simulink model "Simul_ContPID"  (R2024b)
settings: Solver=VariableStepAuto  StartTime=0.0  StopTime=6  RelTol=1e-3
undefined symbols (not defined in the file): Kp, Kpe, T, Te, Ti
settings Model: Creator=Celso  LastModifiedBy=syaba

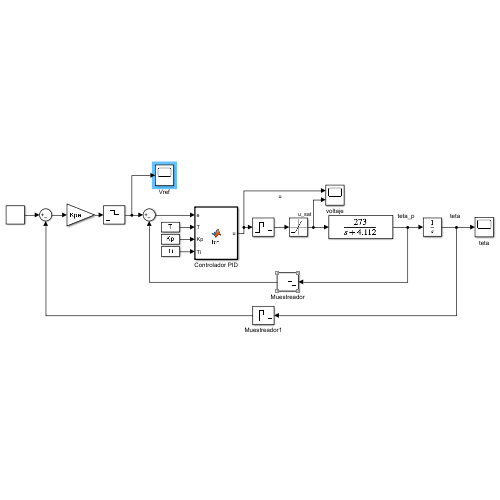
[thumbnail: Simulink's stored preview of the top-level diagram]
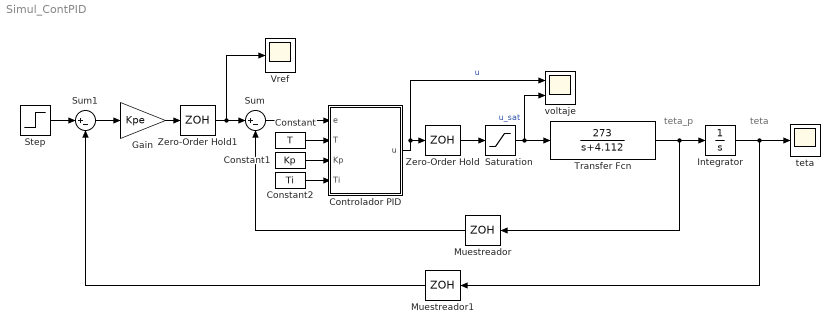
== system Simul_ContPID ==
  note: teta
  note: teta_p
  Constant : Constant  Value=T
  Constant1 : Constant  Value=Kp
  Constant2 : Constant  Value=Ti
  Controlador PID : MATLAB Function  TreatAsAtomicUnit=on  SystemSampleTime=T
  Gain : Gain  Gain=Kpe
  Integrator : Integrator
  Muestreador : ZeroOrderHold  SampleTime=T
  Muestreador1 : ZeroOrderHold  SampleTime=Te
  Saturation : Saturate  UpperLimit=3  LowerLimit=-3
  Step : Step  Time=0  After=100  SampleTime=0
  Sum : Sum  Inputs=|+-
  Sum1 : Sum  Inputs=|+-
  Transfer Fcn : TransferFcn  Numerator=[273]  Denominator=[1 4.112]
  Vref : Scope
  Zero-Order Hold : ZeroOrderHold  SampleTime=T
  Zero-Order Hold1 : ZeroOrderHold  SampleTime=Te
  teta : Scope
  voltaje : Scope  NumInputPorts=2
  wires:
  Constant/1 -> Controlador PID/2(T)
  Sum/1 -> Controlador PID/1(e)
  Controlador PID/1(u) -> voltaje/1, Zero-Order Hold/1  "u"
  Transfer Fcn/1 -> Integrator/1, Muestreador/1
  Muestreador/1 -> Sum/2
  Zero-Order Hold/1 -> Saturation/1
  Saturation/1 -> voltaje/2, Transfer Fcn/1  "u_sat"
  Constant1/1 -> Controlador PID/3(Kp)
  Constant2/1 -> Controlador PID/4(Ti)
  Gain/1 -> Zero-Order Hold1/1
  Zero-Order Hold1/1 -> Vref/1, Sum/1
  Integrator/1 -> teta/1, Muestreador1/1
  Muestreador1/1 -> Sum1/2
  Sum1/1 -> Gain/1
  Step/1 -> Sum1/1

== matlab function Simul_ContPID/Controlador PID ==
  data: e input; u output; T input; Kp input; Ti input
function u = fcn(e,T, Kp, Ti)

persistent I_ant;

if isempty(I_ant),
    I_ant=0;
end;

I = I_ant + e*T;
u = Kp*(e+ (1/Ti)*I);

I_ant = I;
